simulink model "MyPCImages"  (Simulink 7.5)
settings: Solver=FixedStepDiscrete  StartTime=0.0  StopTime=d_data(end,1)  FixedStep=apSampleTime  RelTol=1e-3
InitFcn:
  | replayFlight
values from neighbouring files (symbols this model uses):
  apSampleTime = 0.01    [demoz2SlugsV5.m]
  D = y    [BarOrthog.m]
  R0 = single(Euler2DCMdeg( PHI_IC, THETA_IC, PSI_IC ))    [demoz2SlugsV5.m]
undefined symbols (not defined in the file or in its folder): accBiasRateLimit, accelXCutTemp, axTGain1, axTGain2, axTMean1, axTMean2, barAdjust, baroCutoff, baroCutTemp, baroOffset, baroScale, barTGain1, barTGain2, barTMean1, barTMean2, baseHeight, baseTemp, cubeAccelGain, cubeGyroGain, gaind, GS_location, gyroBiasRateLimit, Init_onlyOnce, Init_Reset, ISA_rho0, lapseRate, lowRateSensorCutoff, magMeanTemp, magOffset, magScale, magTempK, mainSensorCutoff, maxDynPressure, param_acc, param_mag, pitAdjust, pitCutTemp, pitotOffset, pitotScale, pitTGain1, pitTGain2, pitTMean1, pitTMean2, polesd, powerOffset, powerScale, pressureSensorCutoff, T, tempOffset, tempScale, vzCutoff, xCutoff, yCutoff, zCutoff, zerosd
libraries: simulink x11, aerolibconvert2 x9, SLUGS_Library x6, aerolibutil x3, dspmtrx3 x3, dsPICdrivers x1
(part 3 of 4)

== system MyPCImages/Sensor Data/Sensor Suite/Cube Signal Cond/3D Tustin Lowpass, Auto Initial Condition1 ==
  In1 : Inport  OutDataType=sfix(16)  OutScaling=2^0
  Constant : Constant  Value=T  OutDataType=sfix(16)  OutScaling=2^0
  Constant1 : Constant  Value=f  OutDataType=sfix(16)  OutScaling=2^0
  Constant2 : Constant  Value=T  OutDataType=sfix(16)  OutScaling=2^0
  Constant3 : Constant  Value=f  OutDataType=sfix(16)  OutScaling=2^0
  Constant4 : Constant  Value=T  OutDataType=sfix(16)  OutScaling=2^0
  Constant5 : Constant  Value=f  OutDataType=sfix(16)  OutScaling=2^0
  Demux : Demux  Outputs=3
  Embedded MATLAB Function : Stateflow chart  TreatAsAtomicUnit=on
  Embedded MATLAB Function1 : Stateflow chart  TreatAsAtomicUnit=on
  Embedded MATLAB Function2 : Stateflow chart  TreatAsAtomicUnit=on
  myMux Fun : Stateflow chart  TreatAsAtomicUnit=on
  Out1 : Outport  OutDataType=sfix(16)  OutScaling=2^0
  wires:
  Constant/1 -> Embedded MATLAB Function/2(T)
  Constant1/1 -> Embedded MATLAB Function/3(f)
  Embedded MATLAB Function/1(y) -> myMux Fun/1(u1)
  Constant2/1 -> Embedded MATLAB Function1/2(T)
  Constant3/1 -> Embedded MATLAB Function1/3(f)
  Constant4/1 -> Embedded MATLAB Function2/2(T)
  Constant5/1 -> Embedded MATLAB Function2/3(f)
  Embedded MATLAB Function2/1(y) -> myMux Fun/3(u3)
  Demux/1 -> Embedded MATLAB Function/1(u)
  Demux/2 -> Embedded MATLAB Function1/1(u)
  Demux/3 -> Embedded MATLAB Function2/1(u)
  Embedded MATLAB Function1/1(y) -> myMux Fun/2(u2)
  In1/1 -> Demux/1
  myMux Fun/1(y) -> Out1/1

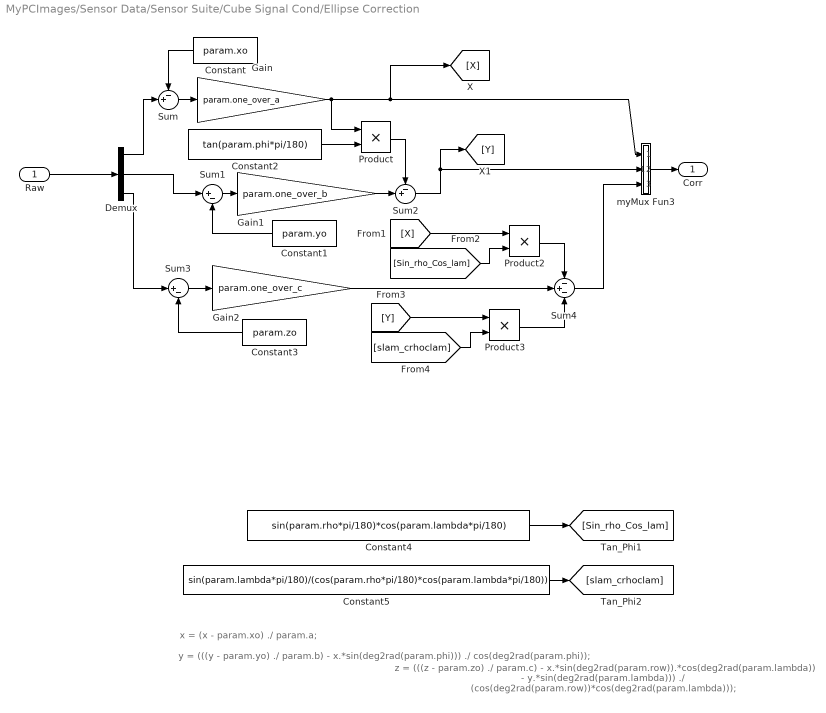
== system MyPCImages/Sensor Data/Sensor Suite/Cube Signal Cond/Ellipse Correction ==
  note: z = (((z - param.zo) ./ param.c) - x.*sin(deg2rad(param.row)).*cos(deg2rad(param.lambda)) - y.*sin(deg2rad(param.lambda))) ./ (cos(deg2rad(param.row))*cos(deg2rad(param.lambda)));
  note: y = (((y - param.yo) ./ param.b) - x.*sin(deg2rad(param.phi))) ./ cos(deg2rad(param.phi));
  note: x = (x - param.xo) ./ param.a;
  Raw : Inport  OutDataType=sfix(16)  OutScaling=2^0
  Constant : Constant  Value=param.xo  OutDataTypeMode=single  OutDataType=sfix(16)  OutScaling=2^0  OutDataTypeStr=single
  Constant1 : Constant  Value=param.yo  OutDataTypeMode=single  OutDataType=sfix(16)  OutScaling=2^0  OutDataTypeStr=single
  Constant2 : Constant  Value=tan(param.phi*pi/180)  OutDataTypeMode=single  OutDataType=sfix(16)  OutScaling=2^0  OutDataTypeStr=single
  Constant3 : Constant  Value=param.zo  OutDataTypeMode=single  OutDataType=sfix(16)  OutScaling=2^0  OutDataTypeStr=single
  Constant4 : Constant  Value=sin(param.rho*pi/180)*cos(param.lambda*pi/180)  OutDataTypeMode=single  OutDataType=sfix(16)  OutScaling=2^0  OutDataTypeStr=single
  Constant5 : Constant  Value=sin(param.lambda*pi/180)/(cos(param.rho*pi/180)*cos(param.lambda*pi/180))  VectorParams1D=off  OutDataTypeMode=single  OutDataType=sfix(16)  OutScaling=2^0  OutDataTypeStr=single
  Demux : Demux  Outputs=3
  Gain : Gain  Gain=param.one_over_a  ParameterDataType=sfix(16)  ParameterScaling=2^0  OutDataType=sfix(16)  OutScaling=2^0
  Gain1 : Gain  Gain=param.one_over_b  ParameterDataType=sfix(16)  ParameterScaling=2^0  OutDataType=sfix(16)  OutScaling=2^0
  Gain2 : Gain  Gain=param.one_over_c  ParameterDataType=sfix(16)  ParameterScaling=2^0  OutDataType=sfix(16)  OutScaling=2^0
  Product : Product  OutDataType=sfix(16)  OutScaling=2^0  RndMeth=Zero
  Product2 : Product  OutDataType=sfix(16)  OutScaling=2^0  RndMeth=Zero
  Product3 : Product  OutDataType=sfix(16)  OutScaling=2^0  RndMeth=Zero
  Sum : Sum  Inputs=-+|  OutDataType=sfix(16)  OutScaling=2^0
  Sum1 : Sum  Inputs=|+-  OutDataType=sfix(16)  OutScaling=2^0
  Sum2 : Sum  Inputs=-+|  OutDataType=sfix(16)  OutScaling=2^0
  Sum3 : Sum  Inputs=|+-  OutDataType=sfix(16)  OutScaling=2^0
  Sum4 : Sum  Inputs=-+-  OutDataType=sfix(16)  OutScaling=2^0
  myMux Fun3 : Stateflow chart  AncestorBlock=SLUGS_Library/Singnal Routing & Conditioning/myMux Fun3  TreatAsAtomicUnit=on
  Corr : Outport  OutDataType=sfix(16)  OutScaling=2^0
  wires:
  Constant5/1 -> [slam_crhoclam]
  Constant4/1 -> [Sin_rho_Cos_lam]
  Sum4/1 -> myMux Fun3/3(u3)
  Product3/1 -> Sum4/3
  [slam_crhoclam] -> Product3/2
  [Y] -> Product3/1
  Product2/1 -> Sum4/1
  [Sin_rho_Cos_lam] -> Product2/2
  [X] -> Product2/1
  Demux/3 -> Sum3/1
  Gain2/1 -> Sum4/2
  Constant3/1 -> Sum3/2
  Sum3/1 -> Gain2/1
  Sum2/1 -> myMux Fun3/2(u2), [Y]
  Product/1 -> Sum2/1
  Gain1/1 -> Sum2/2
  Constant2/1 -> Product/2
  Demux/2 -> Sum1/1
  Constant1/1 -> Sum1/2
  myMux Fun3/1(y) -> Corr/1
  Sum1/1 -> Gain1/1
  Gain/1 -> myMux Fun3/1(u1), Product/1, [X]
  Sum/1 -> Gain/1
  Constant/1 -> Sum/1
  Demux/1 -> Sum/2
  Raw/1 -> Demux/1

== system MyPCImages/Sensor Data/Sensor Suite/Cube Signal Cond/Rotate Cube Axis ==
  Raw : Inport  OutDataType=sfix(16)  OutScaling=2^0
  Selector : Selector  InputPortWidth=3  IndexOptions=Index vector (dialog)  Indices=[2 1 3]  OutputSizes=1
  "[ -1 -1 -1]" : Gain  Gain=[-1 -1 -1]  ParameterDataType=sfix(16)  ParameterScaling=2^0  OutDataType=sfix(16)  OutScaling=2^0
  Rotated : Outport  OutDataType=sfix(16)  OutScaling=2^0
  wires:
  "[ -1 -1 -1]"/1 -> Rotated/1
  Raw/1 -> Selector/1
  Selector/1 -> "[ -1 -1 -1]"/1

== system MyPCImages/Sensor Data/Sensor Suite/Cube Signal Cond/Rotate Cube Axis  ==
  Raw : Inport  OutDataType=sfix(16)  OutScaling=2^0
  Selector : Selector  InputPortWidth=3  IndexOptions=Index vector (dialog)  Indices=[2 1 3]  OutputSizes=1
  Rotated : Outport  OutDataType=sfix(16)  OutScaling=2^0
  wires:
  Selector/1 -> Rotated/1
  Raw/1 -> Selector/1

== system MyPCImages/Sensor Data/Sensor Suite/Cube Signal Cond/Temp Compensate Accel X ==
  Temp : Inport  OutDataType=sfix(16)  OutScaling=2^0
  Accel X : Inport  Port=2  OutDataType=sfix(16)  OutScaling=2^0
  Compare To Constant : simulink/Logic and Bit Operations/Compare To Constant  SystemSampleTime=-1  relop=<  const=accelXCutTemp  LogicOutDataTypeMode=uint8  ZeroCross=off
  Hi Temp Compensation : Subsystem  mask{alpha=axTGain2, tempMean=axTMean2}
      mask prompts: alpha "Tempearature Coeficient (K_t)"; tempMean "Calibration Temperature Mean (T_avg)"
      mask help:
      | This block implements a temperature compensation. It implmements the following equation:
      |
      | M_tc = M_raw - K_t(T - T_avg)
  Lo Temp Compensation : Subsystem  mask{alpha=axTGain1, tempMean=axTMean1}
      mask prompts: alpha "Tempearature Coeficient (K_t)"; tempMean "Calibration Temperature Mean (T_avg)"
      mask help:
      | This block implements a temperature compensation. It implmements the following equation:
      |
      | M_tc = M_raw - K_t(T - T_avg)
  Logical Operator : Logic  Operator=NOT  AllPortsSameDT=off  OutDataTypeMode=boolean  OutDataTypeStr=boolean
  Merge : Merge
  Accel X_c : Outport  OutDataType=sfix(16)  OutScaling=2^0
  wires:
  Logical Operator/1 -> Hi Temp Compensation/Enable
  Merge/1 -> Accel X_c/1
  Lo Temp Compensation/1(Comp) -> Merge/2
  Hi Temp Compensation/1(Comp) -> Merge/1
  Accel X/1 -> Lo Temp Compensation/1(Raw), Hi Temp Compensation/1(Raw)
  Temp/1 -> Lo Temp Compensation/2(Temp Raw), Hi Temp Compensation/2(Temp Raw), Compare To Constant/1
  Compare To Constant/1 -> Lo Temp Compensation/Enable, Logical Operator/1

== system MyPCImages/Sensor Data/Sensor Suite/If no HIL then Read all the Sensors/Accel Raw ==
  Ax1 : FromWorkspace  VariableName=[time ACC_hil(:,1)]  SampleTime=0.01  OutputAfterFinalValue=Setting to zero
  Ay1 : FromWorkspace  VariableName=[time ACC_hil(:,2)]  SampleTime=0.01  OutputAfterFinalValue=Setting to zero
  Az1 : FromWorkspace  VariableName=[time ACC_hil(:,3)]  SampleTime=0.01  OutputAfterFinalValue=Setting to zero
  Data Type Conversion3 : DataTypeConversion  OutDataTypeMode=int16  OutDataType=sfix(16)  OutScaling=2^0  OutDataTypeStr=int16
  Mux1 : Mux  Inputs=3
  Accel : Outport  OutDataType=sfix(16)  OutScaling=2^0
  wires:
  Mux1/1 -> Data Type Conversion3/1
  Ax1/1 -> Mux1/1
  Ay1/1 -> Mux1/2
  Az1/1 -> Mux1/3
  Data Type Conversion3/1 -> Accel/1

== system MyPCImages/Sensor Data/Sensor Suite/If no HIL then Read all the Sensors/Air Data ==
  Baro : FromWorkspace  VariableName=[time STA_hil(:,1)]  SampleTime=0.01  OutputAfterFinalValue=Setting to zero
  COG1 : FromWorkspace  VariableName=[time TEM_hil(:,1)]  SampleTime=0.01  OutputAfterFinalValue=Setting to zero
  Data Type Conversion3 : DataTypeConversion  OutDataTypeMode=uint16  OutDataType=sfix(16)  OutScaling=2^0  OutDataTypeStr=uint16
  Mux1 : Mux
  Pitot : FromWorkspace  VariableName=[time DYN_hil(:,1)]  SampleTime=0.01  OutputAfterFinalValue=Setting to zero
  Power : FromWorkspace  VariableName=[time POW_hil(:,1)]  SampleTime=0.01  OutputAfterFinalValue=Setting to zero
  Air : Outport  OutDataType=sfix(16)  OutScaling=2^0
  wires:
  Baro/1 -> Mux1/1
  Pitot/1 -> Mux1/2
  Power/1 -> Mux1/3
  Mux1/1 -> Data Type Conversion3/1
  COG1/1 -> Mux1/4
  Data Type Conversion3/1 -> Air/1

== system MyPCImages/Sensor Data/Sensor Suite/If no HIL then Read all the Sensors/GPS  ==
  1/100 : Gain  Gain=1/100  ParameterDataType=sfix(16)  ParameterScaling=2^0  OutDataType=sfix(16)  OutScaling=2^0
  COG1 : FromWorkspace  VariableName=[time GPS_hil(:,4)]  SampleTime=0.01  OutputAfterFinalValue=Setting to zero
  Data Type Conversion3 : DataTypeConversion  OutDataTypeMode=single  OutDataType=sfix(16)  OutScaling=2^0  OutDataTypeStr=single
  Hei1 : FromWorkspace  VariableName=[time GPS_hil(:,3)]  SampleTime=0.01  OutputAfterFinalValue=Setting to zero
  Lat1 : FromWorkspace  VariableName=[time GPS_hil(:,1)]  SampleTime=0.01  OutputAfterFinalValue=Setting to zero
  Lon1 : FromWorkspace  VariableName=[time GPS_hil(:,2)]  SampleTime=0.01  OutputAfterFinalValue=Setting to zero
  Mux1 : Mux  Inputs=5
  SOG1 : FromWorkspace  VariableName=[time GPS_hil(:,5)]  SampleTime=0.01  OutputAfterFinalValue=Setting to zero
  GPS : Outport  OutDataType=sfix(16)  OutScaling=2^0
  wires:
  Data Type Conversion3/1 -> GPS/1
  1/100/1 -> Mux1/5
  SOG1/1 -> 1/100/1
  COG1/1 -> Mux1/4
  Mux1/1 -> Data Type Conversion3/1
  Hei1/1 -> Mux1/3
  Lon1/1 -> Mux1/2
  Lat1/1 -> Mux1/1

== system MyPCImages/Sensor Data/Sensor Suite/If no HIL then Read all the Sensors/Gyro Raw ==
  Data Type Conversion3 : DataTypeConversion  OutDataTypeMode=int16  OutDataType=sfix(16)  OutScaling=2^0  OutDataTypeStr=int16
  Mux : Mux  Inputs=3
  p : FromWorkspace  VariableName=[time PQR_hil(:,1)]  SampleTime=0.01  OutputAfterFinalValue=Setting to zero
  q : FromWorkspace  VariableName=[time PQR_hil(:,2)]  SampleTime=0.01  OutputAfterFinalValue=Setting to zero
  r : FromWorkspace  VariableName=[time PQR_hil(:,3)]  SampleTime=0.01  OutputAfterFinalValue=Setting to zero
  Gyro : Outport  OutDataType=sfix(16)  OutScaling=2^0
  wires:
  p/1 -> Mux/1
  q/1 -> Mux/2
  r/1 -> Mux/3
  Mux/1 -> Data Type Conversion3/1
  Data Type Conversion3/1 -> Gyro/1

== system MyPCImages/Sensor Data/Sensor Suite/If no HIL then Read all the Sensors/Mags ==
  Data Type Conversion3 : DataTypeConversion  OutDataTypeMode=int16  OutDataType=sfix(16)  OutScaling=2^0  OutDataTypeStr=int16
  Mux1 : Mux  Inputs=3
  Mx1 : FromWorkspace  VariableName=[time MAG_hil(:,1)]  SampleTime=0.01  OutputAfterFinalValue=Setting to zero
  My1 : FromWorkspace  VariableName=[time MAG_hil(:,2)]  SampleTime=0.01  OutputAfterFinalValue=Setting to zero
  Mz1 : FromWorkspace  VariableName=[time MAG_hil(:,3)]  SampleTime=0.01  OutputAfterFinalValue=Setting to zero
  Mags : Outport  OutDataType=sfix(16)  OutScaling=2^0
  wires:
  Mux1/1 -> Data Type Conversion3/1
  Mz1/1 -> Mux1/3
  My1/1 -> Mux1/2
  Mx1/1 -> Mux1/1
  Data Type Conversion3/1 -> Mags/1

== system MyPCImages/Sensor Data/Sensor Suite/Low Pass Filtering,Temperature Compensation and Calibration/3D Tustin Lowpass, Auto Initial Condition ==
  In1 : Inport  OutDataType=sfix(16)  OutScaling=2^0
  Constant : Constant  Value=T  OutDataType=sfix(16)  OutScaling=2^0
  Constant1 : Constant  Value=f  OutDataType=sfix(16)  OutScaling=2^0
  Constant2 : Constant  Value=T  OutDataType=sfix(16)  OutScaling=2^0
  Constant3 : Constant  Value=f  OutDataType=sfix(16)  OutScaling=2^0
  Constant4 : Constant  Value=T  OutDataType=sfix(16)  OutScaling=2^0
  Constant5 : Constant  Value=f  OutDataType=sfix(16)  OutScaling=2^0
  Demux : Demux  Outputs=3
  Embedded MATLAB Function : Stateflow chart  TreatAsAtomicUnit=on
  Embedded MATLAB Function1 : Stateflow chart  TreatAsAtomicUnit=on
  Embedded MATLAB Function2 : Stateflow chart  TreatAsAtomicUnit=on
  myMux Fun : Stateflow chart  TreatAsAtomicUnit=on
  Out1 : Outport  OutDataType=sfix(16)  OutScaling=2^0
  wires:
  Constant/1 -> Embedded MATLAB Function/2(T)
  Constant1/1 -> Embedded MATLAB Function/3(f)
  Embedded MATLAB Function/1(y) -> myMux Fun/1(u1)
  Constant2/1 -> Embedded MATLAB Function1/2(T)
  Constant3/1 -> Embedded MATLAB Function1/3(f)
  Constant4/1 -> Embedded MATLAB Function2/2(T)
  Constant5/1 -> Embedded MATLAB Function2/3(f)
  Embedded MATLAB Function2/1(y) -> myMux Fun/3(u3)
  Demux/1 -> Embedded MATLAB Function/1(u)
  Demux/2 -> Embedded MATLAB Function1/1(u)
  Demux/3 -> Embedded MATLAB Function2/1(u)
  Embedded MATLAB Function1/1(y) -> myMux Fun/2(u2)
  In1/1 -> Demux/1
  myMux Fun/1(y) -> Out1/1

== system MyPCImages/Sensor Data/Sensor Suite/Low Pass Filtering,Temperature Compensation and Calibration/Baro Altimeter ==
  Static (Pa) : Inport  OutDataType=sfix(16)  OutScaling=2^0
  Compute Barometric Height : Subsystem  mask{baseTemp=baseTemp, LapseRate=lapseRate}
      mask prompts: baseTemp "Base Station Temperature (K)"; LapseRate "Lapse Rate (C/ft)"
      mask help:
      | Produces Altitude in meters from Barometric Pressure in Pascals. Altitude is valid from MSL to 6000 ft.
      |
      | The method implemented here was developed by Ren Curry
  Constant1 : Constant  Value=baseHeight  OutDataTypeMode=single  OutDataType=sfix(16)  OutScaling=2^0  OutDataTypeStr=single
  Enabled Subsystem : Subsystem  TreatAsAtomicUnit=on
  Enables/Disables the Computation of  initial Baro Bias : Stateflow chart  TreatAsAtomicUnit=on
  Initial Baro Bias : Subsystem  TreatAsAtomicUnit=on
  Logical Operator : Logic  Operator=NOT  AllPortsSameDT=off  OutDataTypeMode=boolean  OutDataTypeStr=boolean
  Sum1 : Sum  Inputs=++|  OutDataTypeMode=single  OutDataType=sfix(16)  OutScaling=2^0  OutDataTypeStr=single
  Zero Out Height : Subsystem  TreatAsAtomicUnit=on
  Altitude : Outport  OutDataType=sfix(16)  OutScaling=2^0
  wires:
  Enabled Subsystem/1(Out1) -> Altitude/1
  Sum1/1 -> Enabled Subsystem/1(In1)
  Logical Operator/1 -> Enabled Subsystem/Enable
  Zero Out Height/1(Height Offset) -> Sum1/1
  Initial Baro Bias/1(Baro (Gnd)) -> Compute Barometric Height/2(Base Pressure (Pa))
  Constant1/1 -> Zero Out Height/1(Base Height), Compute Barometric Height/1(Base Height (m))
  Enables/Disables the Computation of  initial Baro Bias/1(tOut) -> Logical Operator/1, Zero Out Height/Enable, Initial Baro Bias/Enable
  Static (Pa)/1 -> Compute Barometric Height/3(Baro (Pa)), Initial Baro Bias/1(Baro (Pa))
  Compute Barometric Height/1("Altitude, m") -> Sum1/2, Zero Out Height/2(Computed Height)

== system MyPCImages/Sensor Data/Sensor Suite/Low Pass Filtering,Temperature Compensation and Calibration/Barometer Unit Conversion ==
  Raw : Inport  OutDataType=sfix(16)  OutScaling=2^0
  Bias : Constant  Value=bias  OutDataTypeMode=single  OutDataType=sfix(16)  OutScaling=2^0  OutDataTypeStr=single
  Divide : Product  OutDataTypeMode=single  OutDataType=sfix(16)  OutScaling=2^-10  OutDataTypeStr=single
  Gains : Constant  Value=gains  OutDataTypeMode=single  OutDataType=sfix(16)  OutScaling=2^0  OutDataTypeStr=single
  Sum : Sum  Inputs=|++  OutDataTypeMode=single  OutDataType=sfix(16)  OutScaling=2^0  OutDataTypeStr=single
  Comp : Outport  OutDataType=sfix(16)  OutScaling=2^0
  wires:
  Sum/1 -> Comp/1
  Divide/1 -> Sum/1
  Gains/1 -> Divide/1
  Raw/1 -> Divide/2
  Bias/1 -> Sum/2

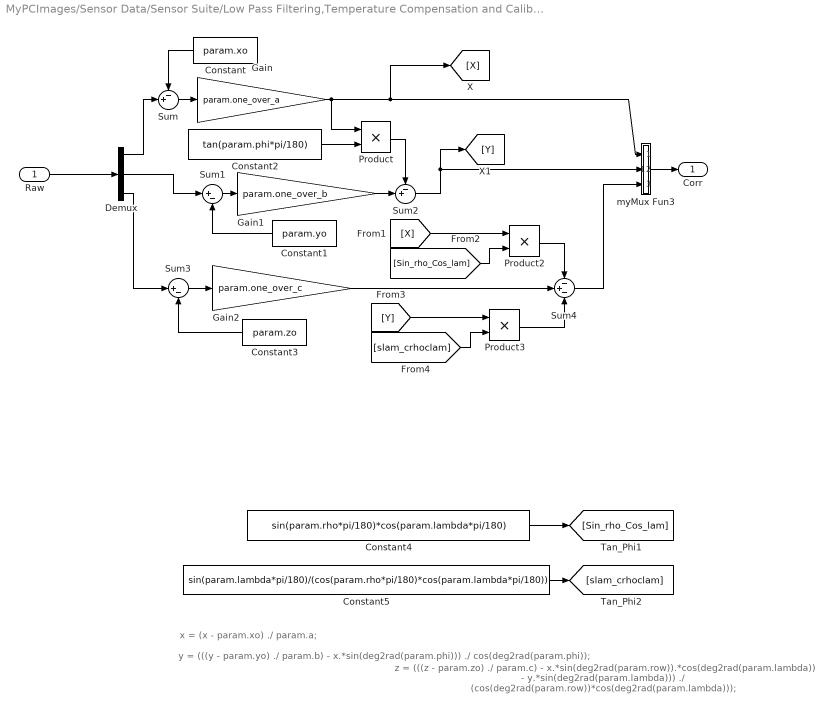
== system MyPCImages/Sensor Data/Sensor Suite/Low Pass Filtering,Temperature Compensation and Calibration/Ellipse Correction ==
  note: z = (((z - param.zo) ./ param.c) - x.*sin(deg2rad(param.row)).*cos(deg2rad(param.lambda)) - y.*sin(deg2rad(param.lambda))) ./ (cos(deg2rad(param.row))*cos(deg2rad(param.lambda)));
  note: y = (((y - param.yo) ./ param.b) - x.*sin(deg2rad(param.phi))) ./ cos(deg2rad(param.phi));
  note: x = (x - param.xo) ./ param.a;
  Raw : Inport  OutDataType=sfix(16)  OutScaling=2^0
  Constant : Constant  Value=param.xo  OutDataTypeMode=single  OutDataType=sfix(16)  OutScaling=2^0  OutDataTypeStr=single
  Constant1 : Constant  Value=param.yo  OutDataTypeMode=single  OutDataType=sfix(16)  OutScaling=2^0  OutDataTypeStr=single
  Constant2 : Constant  Value=tan(param.phi*pi/180)  OutDataTypeMode=single  OutDataType=sfix(16)  OutScaling=2^0  OutDataTypeStr=single
  Constant3 : Constant  Value=param.zo  OutDataTypeMode=single  OutDataType=sfix(16)  OutScaling=2^0  OutDataTypeStr=single
  Constant4 : Constant  Value=sin(param.rho*pi/180)*cos(param.lambda*pi/180)  OutDataTypeMode=single  OutDataType=sfix(16)  OutScaling=2^0  OutDataTypeStr=single
  Constant5 : Constant  Value=sin(param.lambda*pi/180)/(cos(param.rho*pi/180)*cos(param.lambda*pi/180))  VectorParams1D=off  OutDataTypeMode=single  OutDataType=sfix(16)  OutScaling=2^0  OutDataTypeStr=single
  Demux : Demux  Outputs=3
  Gain : Gain  Gain=param.one_over_a  ParameterDataType=sfix(16)  ParameterScaling=2^0  OutDataType=sfix(16)  OutScaling=2^0
  Gain1 : Gain  Gain=param.one_over_b  ParameterDataType=sfix(16)  ParameterScaling=2^0  OutDataType=sfix(16)  OutScaling=2^0
  Gain2 : Gain  Gain=param.one_over_c  ParameterDataType=sfix(16)  ParameterScaling=2^0  OutDataType=sfix(16)  OutScaling=2^0
  Product : Product  OutDataType=sfix(16)  OutScaling=2^0  RndMeth=Zero
  Product2 : Product  OutDataType=sfix(16)  OutScaling=2^0  RndMeth=Zero
  Product3 : Product  OutDataType=sfix(16)  OutScaling=2^0  RndMeth=Zero
  Sum : Sum  Inputs=-+|  OutDataType=sfix(16)  OutScaling=2^0
  Sum1 : Sum  Inputs=|+-  OutDataType=sfix(16)  OutScaling=2^0
  Sum2 : Sum  Inputs=-+|  OutDataType=sfix(16)  OutScaling=2^0
  Sum3 : Sum  Inputs=|+-  OutDataType=sfix(16)  OutScaling=2^0
  Sum4 : Sum  Inputs=-+-  OutDataType=sfix(16)  OutScaling=2^0
  myMux Fun3 : Stateflow chart  AncestorBlock=SLUGS_Library/Singnal Routing & Conditioning/myMux Fun3  TreatAsAtomicUnit=on
  Corr : Outport  OutDataType=sfix(16)  OutScaling=2^0
  wires:
  Constant5/1 -> [slam_crhoclam]
  Constant4/1 -> [Sin_rho_Cos_lam]
  Sum4/1 -> myMux Fun3/3(u3)
  Product3/1 -> Sum4/3
  [slam_crhoclam] -> Product3/2
  [Y] -> Product3/1
  Product2/1 -> Sum4/1
  [Sin_rho_Cos_lam] -> Product2/2
  [X] -> Product2/1
  Demux/3 -> Sum3/1
  Gain2/1 -> Sum4/2
  Constant3/1 -> Sum3/2
  Sum3/1 -> Gain2/1
  Sum2/1 -> myMux Fun3/2(u2), [Y]
  Product/1 -> Sum2/1
  Gain1/1 -> Sum2/2
  Constant2/1 -> Product/2
  Demux/2 -> Sum1/1
  Constant1/1 -> Sum1/2
  myMux Fun3/1(y) -> Corr/1
  Sum1/1 -> Gain1/1
  Gain/1 -> myMux Fun3/1(u1), Product/1, [X]
  Sum/1 -> Gain/1
  Constant/1 -> Sum/1
  Demux/1 -> Sum/2
  Raw/1 -> Demux/1

== system MyPCImages/Sensor Data/Sensor Suite/Low Pass Filtering,Temperature Compensation and Calibration/Magnetometer Unit Conversion ==
  Raw : Inport  OutDataType=sfix(16)  OutScaling=2^0
  Bias : Constant  Value=bias  OutDataTypeMode=single  OutDataType=sfix(16)  OutScaling=2^0  OutDataTypeStr=single
  Divide : Product  OutDataTypeMode=single  OutDataType=sfix(16)  OutScaling=2^-10  OutDataTypeStr=single
  Gains : Constant  Value=gains  OutDataTypeMode=single  OutDataType=sfix(16)  OutScaling=2^0  OutDataTypeStr=single
  Sum : Sum  Inputs=|++  OutDataTypeMode=single  OutDataType=sfix(16)  OutScaling=2^0  OutDataTypeStr=single
  Comp : Outport  OutDataType=sfix(16)  OutScaling=2^0
  wires:
  Sum/1 -> Comp/1
  Divide/1 -> Sum/1
  Gains/1 -> Divide/1
  Raw/1 -> Divide/2
  Bias/1 -> Sum/2

== system MyPCImages/Sensor Data/Sensor Suite/Low Pass Filtering,Temperature Compensation and Calibration/Magnetometers Temp Compensation ==
  Raw : Inport  OutDataType=sfix(16)  OutScaling=2^0
  Temp Raw : Inport  Port=2  OutDataType=sfix(16)  OutScaling=2^0
  Divide1 : Product  OutDataTypeMode=single  OutDataType=sfix(16)  OutScaling=2^-10  OutDataTypeStr=single
  Mean Temperature for Calibration : Constant  Value=tempMean  OutDataTypeMode=single  OutDataType=sfix(16)  OutScaling=2^0  OutDataTypeStr=single
  Sum1 : Sum  Inputs=|+-  OutDataTypeMode=single  OutDataType=sfix(16)  OutScaling=2^0  OutDataTypeStr=single
  Sum2 : Sum  Inputs=|+-  OutDataTypeMode=single  OutDataType=sfix(16)  OutScaling=2^0  OutDataTypeStr=single
  gains : Constant  Value=alpha  OutDataTypeMode=single  OutDataType=sfix(16)  OutScaling=2^0  OutDataTypeStr=single
  Comp : Outport  OutDataType=sfix(16)  OutScaling=2^0
  wires:
  Mean Temperature for Calibration/1 -> Sum1/2
  Raw/1 -> Sum2/1
  Temp Raw/1 -> Sum1/1
  Sum1/1 -> Divide1/2
  gains/1 -> Divide1/1
  Divide1/1 -> Sum2/2
  Sum2/1 -> Comp/1

== system MyPCImages/Sensor Data/Sensor Suite/Low Pass Filtering,Temperature Compensation and Calibration/Pitot Unit Conversion ==
  Raw : Inport  OutDataType=sfix(16)  OutScaling=2^0
  Bias : Constant  Value=bias  OutDataTypeMode=single  OutDataType=sfix(16)  OutScaling=2^0  OutDataTypeStr=single
  Divide : Product  OutDataTypeMode=single  OutDataType=sfix(16)  OutScaling=2^-10  OutDataTypeStr=single
  Gains : Constant  Value=gains  OutDataTypeMode=single  OutDataType=sfix(16)  OutScaling=2^0  OutDataTypeStr=single
  Sum : Sum  Inputs=|++  OutDataTypeMode=single  OutDataType=sfix(16)  OutScaling=2^0  OutDataTypeStr=single
  Comp : Outport  OutDataType=sfix(16)  OutScaling=2^0
  wires:
  Sum/1 -> Comp/1
  Divide/1 -> Sum/1
  Gains/1 -> Divide/1
  Raw/1 -> Divide/2
  Bias/1 -> Sum/2

== system MyPCImages/Sensor Data/Sensor Suite/Low Pass Filtering,Temperature Compensation and Calibration/Power Unit Conversion ==
  Raw : Inport  OutDataType=sfix(16)  OutScaling=2^0
  Bias : Constant  Value=bias  OutDataTypeMode=single  OutDataType=sfix(16)  OutScaling=2^0  OutDataTypeStr=single
  Divide : Product  OutDataTypeMode=single  OutDataType=sfix(16)  OutScaling=2^-10  OutDataTypeStr=single
  Gains : Constant  Value=gains  OutDataTypeMode=single  OutDataType=sfix(16)  OutScaling=2^0  OutDataTypeStr=single
  Sum : Sum  Inputs=|++  OutDataTypeMode=single  OutDataType=sfix(16)  OutScaling=2^0  OutDataTypeStr=single
  Comp : Outport  OutDataType=sfix(16)  OutScaling=2^0
  wires:
  Sum/1 -> Comp/1
  Divide/1 -> Sum/1
  Gains/1 -> Divide/1
  Raw/1 -> Divide/2
  Bias/1 -> Sum/2

== system MyPCImages/Sensor Data/Sensor Suite/Low Pass Filtering,Temperature Compensation and Calibration/Rotate Mags Axis ==
  Raw : Inport  OutDataType=sfix(16)  OutScaling=2^0
  Selector : Selector  InputPortWidth=3  IndexOptions=Index vector (dialog)  Indices=[2 1 3]  OutputSizes=1
  "[ 1 -1 1]" : Gain  Gain=[-1 -1 1]  ParameterDataType=sfix(16)  ParameterScaling=2^0  OutDataType=sfix(16)  OutScaling=2^0
  Rotated : Outport  OutDataType=sfix(16)  OutScaling=2^0
  wires:
  "[ 1 -1 1]"/1 -> Rotated/1
  Raw/1 -> Selector/1
  Selector/1 -> "[ 1 -1 1]"/1

== system MyPCImages/Sensor Data/Sensor Suite/Low Pass Filtering,Temperature Compensation and Calibration/Temp Compensate Accel X1 ==
  Temp : Inport  OutDataType=sfix(16)  OutScaling=2^0
  Dynamic : Inport  Port=2  OutDataType=sfix(16)  OutScaling=2^0
  Compare To Constant : simulink/Logic and Bit Operations/Compare To Constant  SystemSampleTime=-1  relop=<  const=pitCutTemp  LogicOutDataTypeMode=uint8  ZeroCross=off
  Display : Display
  Display2 : Display
  Hi Temp Compensation2 : Subsystem  mask{alpha=pitTGain2, tempMean=pitTMean2}
      mask prompts: alpha "Tempearature Coeficient (K_t)"; tempMean "Calibration Temperature Mean (T_avg)"
      mask help:
      | This block implements a temperature compensation. It implmements the following equation:
      |
      | M_tc = M_raw - K_t(T - T_avg)
  Lo Temp Compensation : Subsystem  mask{alpha=pitTGain1, tempMean=pitTMean1}
      mask prompts: alpha "Tempearature Coeficient (K_t)"; tempMean "Calibration Temperature Mean (T_avg)"
      mask help:
      | This block implements a temperature compensation. It implmements the following equation:
      |
      | M_tc = M_raw - K_t(T - T_avg)
  Logical Operator : Logic  Operator=NOT  AllPortsSameDT=off  OutDataTypeMode=boolean  OutDataTypeStr=boolean
  Merge : Merge
  Baro_c : Outport  OutDataType=sfix(16)  OutScaling=2^0
  wires:
  Lo Temp Compensation/1(Comp) -> Merge/2
  Compare To Constant/1 -> Logical Operator/1, Lo Temp Compensation/Enable
  Temp/1 -> Hi Temp Compensation2/2(Temp Raw), Lo Temp Compensation/2(Temp Raw), Compare To Constant/1
  Dynamic/1 -> Hi Temp Compensation2/1(Raw), Lo Temp Compensation/1(Raw)
  Merge/1 -> Display/1, Baro_c/1
  Logical Operator/1 -> Display2/1, Hi Temp Compensation2/Enable
  Hi Temp Compensation2/1(Comp) -> Merge/1

== system MyPCImages/Sensor Data/Sensor Suite/Low Pass Filtering,Temperature Compensation and Calibration/Temp Compensate Baro ==
  Temp : Inport  OutDataType=sfix(16)  OutScaling=2^0
  Baro : Inport  Port=2  OutDataType=sfix(16)  OutScaling=2^0
  Compare To Constant : simulink/Logic and Bit Operations/Compare To Constant  SystemSampleTime=-1  relop=<  const=baroCutTemp  LogicOutDataTypeMode=uint8  ZeroCross=off
  Hi Temp Compensation : Subsystem  mask{alpha=barTGain2, tempMean=barTMean2}
      mask prompts: alpha "Tempearature Coeficient (K_t)"; tempMean "Calibration Temperature Mean (T_avg)"
      mask help:
      | This block implements a temperature compensation. It implmements the following equation:
      |
      | M_tc = M_raw - K_t(T - T_avg)
  Lo Temp Compensation : Subsystem  mask{alpha=barTGain1, tempMean=barTMean1}
      mask prompts: alpha "Tempearature Coeficient (K_t)"; tempMean "Calibration Temperature Mean (T_avg)"
      mask help:
      | This block implements a temperature compensation. It implmements the following equation:
      |
      | M_tc = M_raw - K_t(T - T_avg)
  Logical Operator : Logic  Operator=NOT  AllPortsSameDT=off  OutDataTypeMode=boolean  OutDataTypeStr=boolean
  Merge : Merge
  Baro_c : Outport  OutDataType=sfix(16)  OutScaling=2^0
  wires:
  Hi Temp Compensation/1(Comp) -> Merge/1
  Logical Operator/1 -> Hi Temp Compensation/Enable
  Merge/1 -> Baro_c/1
  Lo Temp Compensation/1(Comp) -> Merge/2
  Baro/1 -> Lo Temp Compensation/1(Raw), Hi Temp Compensation/1(Raw)
  Temp/1 -> Lo Temp Compensation/2(Temp Raw), Hi Temp Compensation/2(Temp Raw), Compare To Constant/1
  Compare To Constant/1 -> Lo Temp Compensation/Enable, Logical Operator/1

== system MyPCImages/Sensor Data/Sensor Suite/Low Pass Filtering,Temperature Compensation and Calibration/Thermistor Unit Conversion ==
  Raw : Inport  OutDataType=sfix(16)  OutScaling=2^0
  Bias : Constant  Value=bias  OutDataTypeMode=single  OutDataType=sfix(16)  OutScaling=2^0  OutDataTypeStr=single
  Divide : Product  OutDataTypeMode=single  OutDataType=sfix(16)  OutScaling=2^-10  OutDataTypeStr=single
  Gains : Constant  Value=gains  OutDataTypeMode=single  OutDataType=sfix(16)  OutScaling=2^0  OutDataTypeStr=single
  Sum : Sum  Inputs=|++  OutDataTypeMode=single  OutDataType=sfix(16)  OutScaling=2^0  OutDataTypeStr=single
  Comp : Outport  OutDataType=sfix(16)  OutScaling=2^0
  wires:
  Bias/1 -> Sum/2
  Raw/1 -> Divide/2
  Gains/1 -> Divide/1
  Divide/1 -> Sum/1
  Sum/1 -> Comp/1

== system MyPCImages/Sensor Data/Sensor Suite/Low Pass Filtering,Temperature Compensation and Calibration/Tustin Lowpass, Auto Initial Condition1 ==
  In1 : Inport  OutDataType=sfix(16)  OutScaling=2^0
  Constant : Constant  Value=T  OutDataType=sfix(16)  OutScaling=2^0
  Constant1 : Constant  Value=f  OutDataType=sfix(16)  OutScaling=2^0
  Embedded MATLAB Function : Stateflow chart  TreatAsAtomicUnit=on
  Out1 : Outport  OutDataType=sfix(16)  OutScaling=2^0
  wires:
  In1/1 -> Embedded MATLAB Function/1(u)
  Embedded MATLAB Function/1(y) -> Out1/1
  Constant1/1 -> Embedded MATLAB Function/3(f)
  Constant/1 -> Embedded MATLAB Function/2(T)

== system MyPCImages/Sensor Data/Sensor Suite/Low Pass Filtering,Temperature Compensation and Calibration/Tustin Lowpass, Auto Initial Condition2 ==
  In1 : Inport  OutDataType=sfix(16)  OutScaling=2^0
  Constant : Constant  Value=T  OutDataType=sfix(16)  OutScaling=2^0
  Constant1 : Constant  Value=f  OutDataType=sfix(16)  OutScaling=2^0
  Embedded MATLAB Function : Stateflow chart  TreatAsAtomicUnit=on
  Out1 : Outport  OutDataType=sfix(16)  OutScaling=2^0
  wires:
  Constant/1 -> Embedded MATLAB Function/2(T)
  Constant1/1 -> Embedded MATLAB Function/3(f)
  Embedded MATLAB Function/1(y) -> Out1/1
  In1/1 -> Embedded MATLAB Function/1(u)

== system MyPCImages/Sensor Data/Sensor Suite/Low Pass Filtering,Temperature Compensation and Calibration/Tustin Lowpass, Auto Initial Condition3 ==
  In1 : Inport  OutDataType=sfix(16)  OutScaling=2^0
  Constant : Constant  Value=T  OutDataType=sfix(16)  OutScaling=2^0
  Constant1 : Constant  Value=f  OutDataType=sfix(16)  OutScaling=2^0
  Embedded MATLAB Function : Stateflow chart  TreatAsAtomicUnit=on
  Out1 : Outport  OutDataType=sfix(16)  OutScaling=2^0
  wires:
  In1/1 -> Embedded MATLAB Function/1(u)
  Embedded MATLAB Function/1(y) -> Out1/1
  Constant1/1 -> Embedded MATLAB Function/3(f)
  Constant/1 -> Embedded MATLAB Function/2(T)

== system MyPCImages/Sensor Data/Sensor Suite/Low Pass Filtering,Temperature Compensation and Calibration/Tustin Lowpass, Auto Initial Condition4 ==
  In1 : Inport  OutDataType=sfix(16)  OutScaling=2^0
  Constant : Constant  Value=T  OutDataType=sfix(16)  OutScaling=2^0
  Constant1 : Constant  Value=f  OutDataType=sfix(16)  OutScaling=2^0
  Embedded MATLAB Function : Stateflow chart  TreatAsAtomicUnit=on
  Out1 : Outport  OutDataType=sfix(16)  OutScaling=2^0
  wires:
  Constant/1 -> Embedded MATLAB Function/2(T)
  Constant1/1 -> Embedded MATLAB Function/3(f)
  Embedded MATLAB Function/1(y) -> Out1/1
  In1/1 -> Embedded MATLAB Function/1(u)

== system MyPCImages/Sensor Data/Sensor Suite/Low Pass Filtering,Temperature Compensation and Calibration/ValidateMags ==
  In1 : Inport  OutDataType=sfix(16)  OutScaling=2^0
  Hold if Outlier : Subsystem  TreatAsAtomicUnit=on
  Monitor Norm : Subsystem
  Out1 : Outport  OutDataType=sfix(16)  OutScaling=2^0
  wires:
  Hold if Outlier/1(Out1) -> Out1/1
  Monitor Norm/1(Enable) -> Hold if Outlier/Enable
  In1/1 -> Hold if Outlier/1(In1), Monitor Norm/1(Mags)

== system MyPCImages/Position and Attitude Filter/Attitude Complimentary Filter COG/IntegrateGyrosMatrixExp/Rexp, Rodrigues formula/Skew symmetric matrix ==
  omega_in : Inport  OutDataType=fixdt(1, 16)  OutScaling=2^0
  Constant : Constant  Value=0  OutDataType=fixdt(1, 16)  OutScaling=2^0
  Constant1 : Constant  Value=0  OutDataType=fixdt(1, 16)  OutScaling=2^0
  Constant2 : Constant  Value=0  OutDataType=fixdt(1, 16)  OutScaling=2^0
  Demux : Demux  Outputs=3
  Gain : Gain  Gain=-1  ParameterDataType=fixdt(1, 16)  ParameterScaling=2^0  OutDataType=fixdt(1, 16)  OutScaling=2^0
  Gain1 : Gain  Gain=-1  ParameterDataType=fixdt(1, 16)  ParameterScaling=2^0  OutDataType=fixdt(1, 16)  OutScaling=2^0
  Gain2 : Gain  Gain=-1  ParameterDataType=fixdt(1, 16)  ParameterScaling=2^0  OutDataType=fixdt(1, 16)  OutScaling=2^0
  Mux{,1..3} (4 alike) : Mux  Inputs=3
  Reshape : Reshape  OutputDimensionality=Customize  OutputDimensions=[3,3]
  omega_x : Outport  OutDataType=fixdt(1, 16)  OutScaling=2^0
  wires:
  omega_in/1 -> Demux/1
  Reshape/1 -> omega_x/1
  Constant/1 -> Mux/1
  Demux/3 -> Mux/2, Gain1/1
  Demux/2 -> Gain/1, Mux2/1
  Constant1/1 -> Mux1/2
  Demux/1 -> Mux1/3, Gain2/1
  Constant2/1 -> Mux2/3
  Mux/1 -> Mux3/1
  Mux1/1 -> Mux3/2
  Mux2/1 -> Mux3/3
  Mux3/1 -> Reshape/1
  Gain/1 -> Mux/3
  Gain1/1 -> Mux1/1
  Gain2/1 -> Mux2/2

== system MyPCImages/Position and Attitude Filter/Geod2LTP1/ECEF2LTP (UEN)/From Body to Universal1/Rotation Matrix from Long//Lat ==
  note: Calculate Coefficients of DCM Row-Wise
  long lat : Inport  OutDataType=sfix(16)  OutScaling=2^0
  11 : Fcn  Expr=cos(u[1])*cos(u[2])
  12 : Fcn  Expr=sin(u[1])*cos(u[2])
  13 : Fcn  Expr=sin(u[2])
  21 : Fcn  Expr=-sin(u[1])
  22 : Fcn  Expr=cos(u[1])
  23 : Fcn  Expr=0
  31 : Fcn  Expr=-sin(u[2])*cos(u[1])
  32 : Fcn  Expr=-sin(u[1])*sin(u[2])
  33 : Fcn  Expr=cos(u[2])
  Mux2 : Mux  Inputs=9
  DCM : Outport  OutDataType=sfix(16)  OutScaling=2^0  InitialOutput=0
  wires:
  33/1 -> Mux2/9
  23/1 -> Mux2/8
  13/1 -> Mux2/7
  32/1 -> Mux2/6
  22/1 -> Mux2/5
  12/1 -> Mux2/4
  31/1 -> Mux2/3
  21/1 -> Mux2/2
  11/1 -> Mux2/1
  Mux2/1 -> DCM/1
  long lat/1 -> 11/1, 33/1, 23/1, 13/1, 32/1, 22/1, 12/1, 31/1, 21/1

== system MyPCImages/Position and Attitude Filter/Position Filter/BlendPosVel/1D Filter/Filter2 ==
  In1 : Inport  OutDataType=sfix(16)  OutScaling=2^0
  Discrete Zero-Pole : DiscreteZeroPole  Zeros=zerosd  Poles=polesd  Gain=gaind  SampleTime=SampleTime
  Out1 : Outport  OutDataType=sfix(16)  OutScaling=2^0
  wires:
  Discrete Zero-Pole/1 -> Out1/1
  In1/1 -> Discrete Zero-Pole/1

== system MyPCImages/Position and Attitude Filter/Position Filter/BlendPosVel/1D Filter2/Filter2 ==
  In1 : Inport  OutDataType=sfix(16)  OutScaling=2^0
  Discrete Zero-Pole : DiscreteZeroPole  Zeros=zerosd  Poles=polesd  Gain=gaind  SampleTime=SampleTime
  Out1 : Outport  OutDataType=sfix(16)  OutScaling=2^0
  wires:
  Discrete Zero-Pole/1 -> Out1/1
  In1/1 -> Discrete Zero-Pole/1

== system MyPCImages/Position and Attitude Filter/Position Filter/BlendPosVel/2 FIlter Blend/1D Filter ==
  In1 : Inport  OutDataType=sfix(16)  OutScaling=2^0
  Data Type Conversion1 : DataTypeConversion  OutDataTypeMode=single  OutDataType=sfix(16)  OutScaling=2^0  OutDataTypeStr=single
  Data Type Conversion2 : DataTypeConversion  OutDataTypeMode=double  OutDataType=sfix(16)  OutScaling=2^0  OutDataTypeStr=double
  Filter2 : Subsystem  mask(DiscretizedZeroPole){Zeros=zval, Poles=pval, Gain=kval, AbsTol=auto, SampleTime=TSample, method=tustin, Wc=1}
      mask prompts: Zeros "Zeros (enter in s-main:)"; Poles "Poles (enter in s-domain:)"; Gain "Gain (enter in s-domain:)"; AbsTol "Absolute tolerance:"; SampleTime "Sample time:"; Wc "Critical Frequency (Hz):"
      mask help: Continuous mask uses c2d to transform parameters onto the Discrete Zero-Pole block inside.
      mask init: same as MyPCImages/Position and Attitude Filter/Attitude Complimentary Filter COG/3D Filter/Filter1
      mask StyleString: edit,edit,edit,edit,edit,popup(zoh|foh|tustin|prewarp|matched),edit
      mask CallbackString: |||||hidecrit|
      mask Display:
      | droots(zeross,poless,gainss)
      | text( 0.5, 1.0, method, 'verticalAlignment','top')
  Out1 : Outport  OutDataType=sfix(16)  OutScaling=2^0
  wires:
  Data Type Conversion1/1 -> Out1/1
  Data Type Conversion2/1 -> Filter2/1(In1)
  In1/1 -> Data Type Conversion2/1
  Filter2/1(Out1) -> Data Type Conversion1/1

== system MyPCImages/Position and Attitude Filter/Position Filter/BlendPosVel/2 FIlter Blend/1D Filter1 ==
  In1 : Inport  OutDataType=sfix(16)  OutScaling=2^0
  Data Type Conversion1 : DataTypeConversion  OutDataTypeMode=single  OutDataType=sfix(16)  OutScaling=2^0  OutDataTypeStr=single
  Data Type Conversion2 : DataTypeConversion  OutDataTypeMode=double  OutDataType=sfix(16)  OutScaling=2^0  OutDataTypeStr=double
  Filter2 : Subsystem  mask(DiscretizedZeroPole){Zeros=zval, Poles=pval, Gain=kval, AbsTol=auto, SampleTime=TSample, method=tustin, Wc=1}
      mask prompts: Zeros "Zeros (enter in s-main:)"; Poles "Poles (enter in s-domain:)"; Gain "Gain (enter in s-domain:)"; AbsTol "Absolute tolerance:"; SampleTime "Sample time:"; Wc "Critical Frequency (Hz):"
      mask help: Continuous mask uses c2d to transform parameters onto the Discrete Zero-Pole block inside.
      mask init: same as MyPCImages/Position and Attitude Filter/Attitude Complimentary Filter COG/3D Filter/Filter1
      mask StyleString: edit,edit,edit,edit,edit,popup(zoh|foh|tustin|prewarp|matched),edit
      mask CallbackString: |||||hidecrit|
      mask Display:
      | droots(zeross,poless,gainss)
      | text( 0.5, 1.0, method, 'verticalAlignment','top')
  Out1 : Outport  OutDataType=sfix(16)  OutScaling=2^0
  wires:
  Filter2/1(Out1) -> Data Type Conversion1/1
  In1/1 -> Data Type Conversion2/1
  Data Type Conversion2/1 -> Filter2/1(In1)
  Data Type Conversion1/1 -> Out1/1

== system MyPCImages/Position and Attitude Filter/Position Filter/BlendPosVel/3D Filter/Filter1 ==
  In1 : Inport  OutDataType=sfix(16)  OutScaling=2^0
  Discrete Zero-Pole : DiscreteZeroPole  Zeros=zerosd  Poles=polesd  Gain=gaind  SampleTime=SampleTime
  Out1 : Outport  OutDataType=sfix(16)  OutScaling=2^0
  wires:
  In1/1 -> Discrete Zero-Pole/1
  Discrete Zero-Pole/1 -> Out1/1

== system MyPCImages/Position and Attitude Filter/Position Filter/BlendPosVel/3D Filter/Filter2 ==
  In1 : Inport  OutDataType=sfix(16)  OutScaling=2^0
  Discrete Zero-Pole : DiscreteZeroPole  Zeros=zerosd  Poles=polesd  Gain=gaind  SampleTime=SampleTime
  Out1 : Outport  OutDataType=sfix(16)  OutScaling=2^0
  wires:
  Discrete Zero-Pole/1 -> Out1/1
  In1/1 -> Discrete Zero-Pole/1

== system MyPCImages/Position and Attitude Filter/Position Filter/BlendPosVel/3D Filter/Filter3 ==
  In1 : Inport  OutDataType=sfix(16)  OutScaling=2^0
  Discrete Zero-Pole : DiscreteZeroPole  Zeros=zerosd  Poles=polesd  Gain=gaind  SampleTime=SampleTime
  Out1 : Outport  OutDataType=sfix(16)  OutScaling=2^0
  wires:
  In1/1 -> Discrete Zero-Pole/1
  Discrete Zero-Pole/1 -> Out1/1

== system MyPCImages/Position and Attitude Filter/Position Filter/BlendPosVel/CompFiltRate/1D Filter1 ==
  In1 : Inport  OutDataType=sfix(16)  OutScaling=2^0
  Data Type Conversion1 : DataTypeConversion  OutDataTypeMode=single  OutDataType=sfix(16)  OutScaling=2^0  OutDataTypeStr=single
  Data Type Conversion2 : DataTypeConversion  OutDataTypeMode=double  OutDataType=sfix(16)  OutScaling=2^0  OutDataTypeStr=double
  Filter2 : Subsystem  mask(DiscretizedZeroPole){Zeros=zval, Poles=pval, Gain=kval, AbsTol=auto, SampleTime=TSample, method=tustin, Wc=1}
      mask prompts: Zeros "Zeros (enter in s-main:)"; Poles "Poles (enter in s-domain:)"; Gain "Gain (enter in s-domain:)"; AbsTol "Absolute tolerance:"; SampleTime "Sample time:"; Wc "Critical Frequency (Hz):"
      mask help: Continuous mask uses c2d to transform parameters onto the Discrete Zero-Pole block inside.
      mask init: same as MyPCImages/Position and Attitude Filter/Attitude Complimentary Filter COG/3D Filter/Filter1
      mask StyleString: edit,edit,edit,edit,edit,popup(zoh|foh|tustin|prewarp|matched),edit
      mask CallbackString: |||||hidecrit|
      mask Display:
      | droots(zeross,poless,gainss)
      | text( 0.5, 1.0, method, 'verticalAlignment','top')
  Out1 : Outport  OutDataType=sfix(16)  OutScaling=2^0
  wires:
  Filter2/1(Out1) -> Data Type Conversion1/1
  In1/1 -> Data Type Conversion2/1
  Data Type Conversion2/1 -> Filter2/1(In1)
  Data Type Conversion1/1 -> Out1/1

== system MyPCImages/Position and Attitude Filter/Position Filter/BlendPosVel/CompFiltRate1/1D Filter1 ==
  In1 : Inport  OutDataType=sfix(16)  OutScaling=2^0
  Data Type Conversion1 : DataTypeConversion  OutDataTypeMode=single  OutDataType=sfix(16)  OutScaling=2^0  OutDataTypeStr=single
  Data Type Conversion2 : DataTypeConversion  OutDataTypeMode=double  OutDataType=sfix(16)  OutScaling=2^0  OutDataTypeStr=double
  Filter2 : Subsystem  mask(DiscretizedZeroPole){Zeros=zval, Poles=pval, Gain=kval, AbsTol=auto, SampleTime=TSample, method=tustin, Wc=1}
      mask prompts: Zeros "Zeros (enter in s-main:)"; Poles "Poles (enter in s-domain:)"; Gain "Gain (enter in s-domain:)"; AbsTol "Absolute tolerance:"; SampleTime "Sample time:"; Wc "Critical Frequency (Hz):"
      mask help: Continuous mask uses c2d to transform parameters onto the Discrete Zero-Pole block inside.
      mask init: same as MyPCImages/Position and Attitude Filter/Attitude Complimentary Filter COG/3D Filter/Filter1
      mask StyleString: edit,edit,edit,edit,edit,popup(zoh|foh|tustin|prewarp|matched),edit
      mask CallbackString: |||||hidecrit|
      mask Display:
      | droots(zeross,poless,gainss)
      | text( 0.5, 1.0, method, 'verticalAlignment','top')
  Out1 : Outport  OutDataType=sfix(16)  OutScaling=2^0
  wires:
  Filter2/1(Out1) -> Data Type Conversion1/1
  In1/1 -> Data Type Conversion2/1
  Data Type Conversion2/1 -> Filter2/1(In1)
  Data Type Conversion1/1 -> Out1/1

== system MyPCImages/Position and Attitude Filter/Position Filter/BlendPosVel/CompRateOnly/1D Filter1 ==
  In1 : Inport  OutDataType=sfix(16)  OutScaling=2^0
  Data Type Conversion1 : DataTypeConversion  OutDataTypeMode=single  OutDataType=sfix(16)  OutScaling=2^0  OutDataTypeStr=single
  Data Type Conversion2 : DataTypeConversion  OutDataTypeMode=double  OutDataType=sfix(16)  OutScaling=2^0  OutDataTypeStr=double
  Filter2 : Subsystem  mask(DiscretizedZeroPole){Zeros=zval, Poles=pval, Gain=kval, AbsTol=auto, SampleTime=TSample, method=tustin, Wc=1}
      mask prompts: Zeros "Zeros (enter in s-main:)"; Poles "Poles (enter in s-domain:)"; Gain "Gain (enter in s-domain:)"; AbsTol "Absolute tolerance:"; SampleTime "Sample time:"; Wc "Critical Frequency (Hz):"
      mask help: Continuous mask uses c2d to transform parameters onto the Discrete Zero-Pole block inside.
      mask init: same as MyPCImages/Position and Attitude Filter/Attitude Complimentary Filter COG/3D Filter/Filter1
      mask StyleString: edit,edit,edit,edit,edit,popup(zoh|foh|tustin|prewarp|matched),edit
      mask CallbackString: |||||hidecrit|
      mask Display:
      | droots(zeross,poless,gainss)
      | text( 0.5, 1.0, method, 'verticalAlignment','top')
  Out1 : Outport  OutDataType=sfix(16)  OutScaling=2^0
  wires:
  Filter2/1(Out1) -> Data Type Conversion1/1
  In1/1 -> Data Type Conversion2/1
  Data Type Conversion2/1 -> Filter2/1(In1)
  Data Type Conversion1/1 -> Out1/1

== system MyPCImages/Sensor Data/Sensor Suite/Cube Signal Cond/Temp Compensate Accel X/Hi Temp Compensation ==
  Raw : Inport  OutDataType=sfix(16)  OutScaling=2^0
  Temp Raw : Inport  Port=2  OutDataType=sfix(16)  OutScaling=2^0
  Enable : EnablePort
  Divide1 : Product  OutDataTypeMode=single  OutDataType=sfix(16)  OutScaling=2^-10  OutDataTypeStr=single
  Mean Temperature for Calibration : Constant  Value=tempMean  OutDataTypeMode=single  OutDataType=sfix(16)  OutScaling=2^0  OutDataTypeStr=single
  Sum1 : Sum  Inputs=|+-  OutDataTypeMode=single  OutDataType=sfix(16)  OutScaling=2^0  OutDataTypeStr=single
  Sum2 : Sum  Inputs=|+-  OutDataTypeMode=single  OutDataType=sfix(16)  OutScaling=2^0  OutDataTypeStr=single
  gains : Constant  Value=alpha  OutDataTypeMode=single  OutDataType=sfix(16)  OutScaling=2^0  OutDataTypeStr=single
  Comp : Outport  OutDataType=sfix(16)  OutScaling=2^0
  wires:
  Mean Temperature for Calibration/1 -> Sum1/2
  Raw/1 -> Sum2/1
  Temp Raw/1 -> Sum1/1
  Sum1/1 -> Divide1/2
  gains/1 -> Divide1/1
  Divide1/1 -> Sum2/2
  Sum2/1 -> Comp/1

== system MyPCImages/Sensor Data/Sensor Suite/Cube Signal Cond/Temp Compensate Accel X/Lo Temp Compensation ==
  Raw : Inport  OutDataType=sfix(16)  OutScaling=2^0
  Temp Raw : Inport  Port=2  OutDataType=sfix(16)  OutScaling=2^0
  Enable : EnablePort
  Divide1 : Product  OutDataTypeMode=single  OutDataType=sfix(16)  OutScaling=2^-10  OutDataTypeStr=single
  Mean Temperature for Calibration : Constant  Value=tempMean  OutDataTypeMode=single  OutDataType=sfix(16)  OutScaling=2^0  OutDataTypeStr=single
  Sum1 : Sum  Inputs=|+-  OutDataTypeMode=single  OutDataType=sfix(16)  OutScaling=2^0  OutDataTypeStr=single
  Sum2 : Sum  Inputs=|+-  OutDataTypeMode=single  OutDataType=sfix(16)  OutScaling=2^0  OutDataTypeStr=single
  gains : Constant  Value=alpha  OutDataTypeMode=single  OutDataType=sfix(16)  OutScaling=2^0  OutDataTypeStr=single
  Comp : Outport  OutDataType=sfix(16)  OutScaling=2^0
  wires:
  Sum2/1 -> Comp/1
  Divide1/1 -> Sum2/2
  gains/1 -> Divide1/1
  Sum1/1 -> Divide1/2
  Temp Raw/1 -> Sum1/1
  Raw/1 -> Sum2/1
  Mean Temperature for Calibration/1 -> Sum1/2

== system MyPCImages/Sensor Data/Sensor Suite/Low Pass Filtering,Temperature Compensation and Calibration/Baro Altimeter/Compute Barometric Height ==
  Base Height (m) : Inport  OutDataType=sfix(16)  OutScaling=2^0
  Base Pressure (Pa) : Inport  Port=2  OutDataType=sfix(16)  OutScaling=2^0
  Baro (Pa) : Inport  Port=3  OutDataType=sfix(16)  OutScaling=2^0
  Constant2 : Constant  Value=baseTemp/(-LapseRate)  OutDataTypeMode=single  OutDataType=sfix(16)  OutScaling=2^0  OutDataTypeStr=single
  Constant3 : Constant  Value=9.350253e-2  OutDataTypeMode=single  OutDataType=sfix(16)  OutScaling=2^0  OutDataTypeStr=single
  Constant4 : Constant  Value=-1.888933e-1  OutDataTypeMode=single  OutDataType=sfix(16)  OutScaling=2^0  OutDataTypeStr=single
  Constant5 : Constant  Value=2.180313e-5  OutDataTypeMode=single  OutDataType=sfix(16)  OutScaling=2^0  OutDataTypeStr=single
  Divide : Product  Inputs=*/  OutDataTypeMode=single  OutDataType=sfix(16)  OutScaling=2^-10  OutDataTypeStr=single
  Divide{1..4} (4 alike) : Product  OutDataTypeMode=single  OutDataType=sfix(16)  OutScaling=2^-10  OutDataTypeStr=single
  Length Conversion : aerolibconvert2/Length Conversion  SystemSampleTime=-1  IU=ft  OU=m
  Sum1 : Sum  Inputs=|++  OutDataTypeMode=single  OutDataType=sfix(16)  OutScaling=2^0  OutDataTypeStr=single
  Sum2 : Sum  Inputs=|+-  OutDataTypeMode=single  OutDataType=sfix(16)  OutScaling=2^0  OutDataTypeStr=single
  Sum3 : Sum  Inputs=3  OutDataTypeMode=single  OutDataType=sfix(16)  OutScaling=2^0  OutDataTypeStr=single
  "Altitude, m" : Outport  OutDataType=sfix(16)  OutScaling=2^0
  wires:
  Baro (Pa)/1 -> Sum2/1
  Base Height (m)/1 -> Sum1/2
  Base Pressure (Pa)/1 -> Sum2/2, Divide/2
  Divide/1 -> Divide4/2, Divide4/1, Divide2/1  "x"
  Divide4/1 -> Divide1/1  "x^2"
  Constant3/1 -> Divide1/2
  Constant4/1 -> Divide2/2
  Divide1/1 -> Sum3/1
  Divide2/1 -> Sum3/2
  Constant5/1 -> Sum3/3
  Sum3/1 -> Divide3/1
  Constant2/1 -> Divide3/2
  Divide3/1 -> Length Conversion/1
  Sum1/1 -> "Altitude, m"/1
  Sum2/1 -> Divide/1
  Length Conversion/1 -> Sum1/1

== system MyPCImages/Sensor Data/Sensor Suite/Low Pass Filtering,Temperature Compensation and Calibration/Baro Altimeter/Enabled Subsystem ==
  In1 : Inport  OutDataType=sfix(16)  OutScaling=2^0
  Enable : EnablePort
  Out1 : Outport  OutDataType=sfix(16)  OutScaling=2^0  InitialOutput=baseHeight
  wires:
  In1/1 -> Out1/1

== system MyPCImages/Sensor Data/Sensor Suite/Low Pass Filtering,Temperature Compensation and Calibration/Baro Altimeter/Initial Baro Bias ==
  Baro (Pa) : Inport  OutDataType=sfix(16)  OutScaling=2^0
  Enable : EnablePort
  Data Type Conversion : DataTypeConversion  OutDataTypeMode=double  OutDataType=sfix(16)  OutScaling=2^0  OutDataTypeStr=double
  Data Type Conversion1 : DataTypeConversion  OutDataTypeMode=single  OutDataType=sfix(16)  OutScaling=2^0  OutDataTypeStr=single
  Low Pass8 : Subsystem  mask(DiscretizedZeroPole){Zeros=[], Poles=[-3], Gain=3, AbsTol=auto, SampleTime=.01, method=tustin, Wc=1}
      mask prompts: Zeros "Zeros (enter in s-main:)"; Poles "Poles (enter in s-domain:)"; Gain "Gain (enter in s-domain:)"; AbsTol "Absolute tolerance:"; SampleTime "Sample time:"; Wc "Critical Frequency (Hz):"
      mask help: Continuous mask uses c2d to transform parameters onto the Discrete Zero-Pole block inside.
      mask init: same as MyPCImages/Position and Attitude Filter/Attitude Complimentary Filter COG/3D Filter/Filter1
      mask StyleString: edit,edit,edit,edit,edit,popup(zoh|foh|tustin|prewarp|matched),edit
      mask CallbackString: |||||hidecrit|
      mask Display:
      | droots(zeross,poless,gainss)
      | text( 0.5, 1.0, method, 'verticalAlignment','top')
  Mux : Mux  Inputs=2
  Scope : Scope
      settings: SaveName=ScopeData8
  "[80k - 120k]" : Saturate  UpperLimit=120000  LowerLimit=80000
  Baro (Gnd) : Outport  OutDataType=sfix(16)  OutScaling=2^0
  wires:
  "[80k - 120k]"/1 -> Mux/1, Baro (Gnd)/1
  Mux/1 -> Scope/1
  Data Type Conversion1/1 -> "[80k - 120k]"/1, Mux/2
  Data Type Conversion/1 -> Low Pass8/1(In1)
  Low Pass8/1(Out1) -> Data Type Conversion1/1
  Baro (Pa)/1 -> Data Type Conversion/1
